simulink model "NandiniG_23EEM1S02_foc_5mli_working_fine_Cap"  (R2024b)
settings: Solver=ode1  StartTime=0.0  StopTime=1  FixedStep=0.000001  MaxStep=1e-4  RelTol=1e-3
model workspace (MAT data in the model file):
  Vdcref = 40
  Vref = 450
  fs = 2054
  k = 1
  ma = 1
undefined symbols (not defined in the file): Kcq, Kcs
libraries: spsIGBTDiodeLib x28, simulink x20, spsDiodeLib x18, spsVoltageMeasurementLib x12, slpidlib x9, spsSeriesRLCBranchLib x8, powerlib_extras x3, spsCurrentMeasurementLib x3, spsDCVoltageSourceLib x1, spsGroundLib x1, spsPermanentMagnetSynchronousMachineLib x1, spsThreePhaseVIMeasurementLib x1
(part 2 of 2)

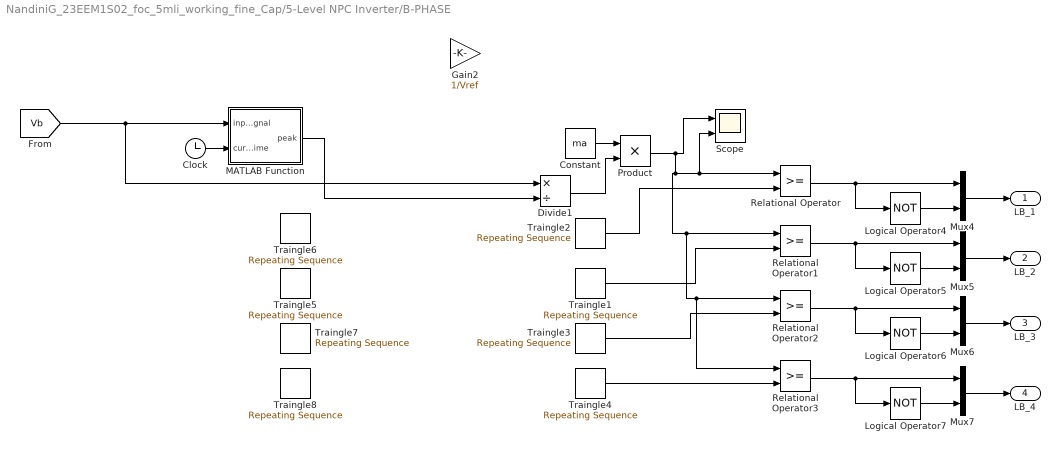
== system NandiniG_23EEM1S02_foc_5mli_working_fine_Cap/5-Level NPC Inverter/B-PHASE ==
  Clock : Clock
  Constant : Constant  Value=ma
  Divide1 : Product  Inputs=*/
  Gain2 : Gain  Gain=1/Vref
  Logical Operator{4..7} (4 alike) : Logic  Operator=NOT  AllPortsSameDT=off  OutDataTypeStr=boolean
  MATLAB Function : MATLAB Function  TreatAsAtomicUnit=on
  Mux{4..7} (4 alike) : Mux  Inputs=2
  Product : Product
  Relational Operator{,1..3} (4 alike) : RelationalOperator  OutDataTypeStr=boolean  InputSameDT=off
  Scope : Scope  NumInputPorts=2
  Traingle1 : simulink/Sources/Repeating Sequence  rep_seq_t=[0 0.25/fs 0.5/fs 0.75/fs 1/fs]  rep_seq_y=[0 0.25 0.5 0.25 0]*k
  Traingle2 : simulink/Sources/Repeating Sequence  rep_seq_t=[0 0.25/fs 0.5/fs 0.75/fs 1/fs]  rep_seq_y="[0.5 0.75 1 0.75  0.5]*k"
  Traingle3 : simulink/Sources/Repeating Sequence  rep_seq_t=[0 0.25/fs 0.5/fs 0.75/fs 1/fs]  rep_seq_y=[-0.5 -0.25 0 -0.25 -0.5]*k
  Traingle4 : simulink/Sources/Repeating Sequence  rep_seq_t=[0 0.25/fs 0.5/fs 0.75/fs 1/fs]  rep_seq_y=[-1 -0.75 -0.5 -0.75 -1]*k
  Traingle5 : simulink/Sources/Repeating Sequence  rep_seq_t=[0 0.25/fs 0.5/fs 0.75/fs 1/fs]  rep_seq_y=[565*0.25 565/2 565*0.25 0 565*0.25]
  Traingle6 : simulink/Sources/Repeating Sequence  rep_seq_t=[0 0.25/fs 0.5/fs 0.75/fs 1/fs]  rep_seq_y=[565*0.75 565 565*0.75 565/2 565*0.75]
  Traingle7 : simulink/Sources/Repeating Sequence  rep_seq_t=[0 0.25/fs 0.5/fs 0.75/fs 1/fs]  rep_seq_y=[-565*0.25 0 -565*0.25 -565/2 -565*0.25]
  Traingle8 : simulink/Sources/Repeating Sequence  rep_seq_t=[0 0.25/fs 0.5/fs 0.75/fs 1/fs]  rep_seq_y=[-565*0.75 -565/2 -565*0.75 -565 -565*0.75]
  LB_1 : Outport
  LB_2 : Outport  Port=2
  LB_3 : Outport  Port=3
  LB_4 : Outport  Port=4
  wires:
  Relational Operator/1 -> Logical Operator4/1, Mux4/1
  Logical Operator4/1 -> Mux4/2
  Mux4/1 -> LB_1/1
  Relational Operator1/1 -> Mux5/1, Logical Operator5/1
  Logical Operator5/1 -> Mux5/2
  Mux5/1 -> LB_2/1
  Relational Operator2/1 -> Logical Operator6/1, Mux6/1
  Logical Operator6/1 -> Mux6/2
  Mux6/1 -> LB_3/1
  Relational Operator3/1 -> Mux7/1, Logical Operator7/1
  Logical Operator7/1 -> Mux7/2
  Mux7/1 -> LB_4/1
  Traingle1/1 -> Relational Operator1/2
  Traingle2/1 -> Relational Operator/2
  Traingle4/1 -> Relational Operator3/2
  Traingle3/1 -> Relational Operator2/2
  [Vb] -> MATLAB Function/1(inputSignal), Divide1/1
  MATLAB Function/1(peak) -> Divide1/2
  Divide1/1 -> Product/2
  Constant/1 -> Product/1
  Product/1 -> Relational Operator3/1, Relational Operator2/1, Relational Operator1/1, Scope/2, Relational Operator/1, Scope/1
  Clock/1 -> MATLAB Function/2(currentTime)

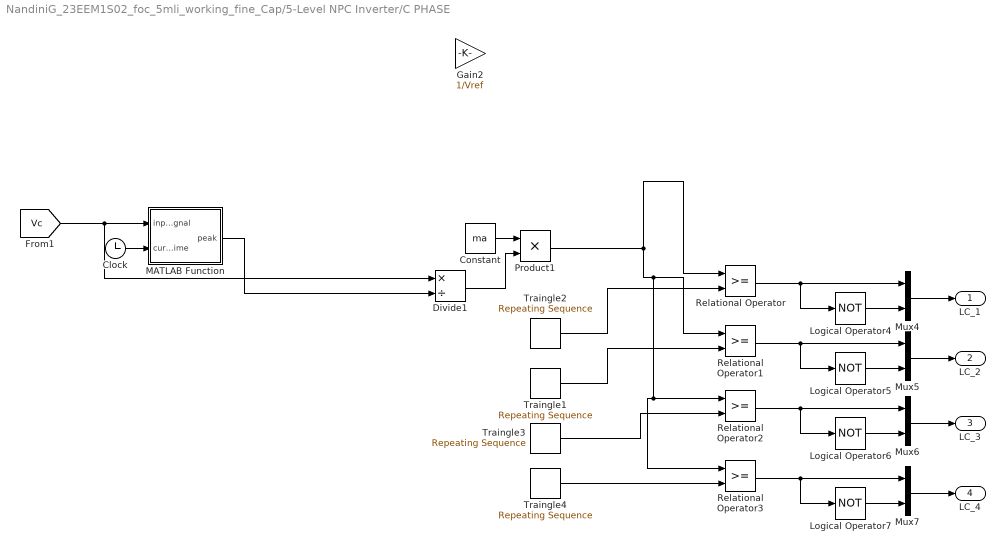
== system NandiniG_23EEM1S02_foc_5mli_working_fine_Cap/5-Level NPC Inverter/C PHASE ==
  Clock : Clock
  Constant : Constant  Value=ma
  Divide1 : Product  Inputs=*/
  Gain2 : Gain  Gain=1/Vref
  Logical Operator{4..7} (4 alike) : Logic  Operator=NOT  AllPortsSameDT=off  OutDataTypeStr=boolean
  MATLAB Function : MATLAB Function  TreatAsAtomicUnit=on
  Mux{4..7} (4 alike) : Mux  Inputs=2
  Product1 : Product
  Relational Operator{,1..3} (4 alike) : RelationalOperator  OutDataTypeStr=boolean  InputSameDT=off
  Traingle1 : simulink/Sources/Repeating Sequence  rep_seq_t=[0 0.25/fs 0.5/fs 0.75/fs 1/fs]  rep_seq_y=[0 0.25 0.5 0.25 0]*k
  Traingle2 : simulink/Sources/Repeating Sequence  rep_seq_t=[0 0.25/fs 0.5/fs 0.75/fs 1/fs]  rep_seq_y="[0.5 0.75 1 0.75  0.5]*k"
  Traingle3 : simulink/Sources/Repeating Sequence  rep_seq_t=[0 0.25/fs 0.5/fs 0.75/fs 1/fs]  rep_seq_y=[-0.5 -0.25 0 -0.25 -0.5]*k
  Traingle4 : simulink/Sources/Repeating Sequence  rep_seq_t=[0 0.25/fs 0.5/fs 0.75/fs 1/fs]  rep_seq_y=[-1 -0.75 -0.5 -0.75 -1]*k
  LC_1 : Outport
  LC_2 : Outport  Port=2
  LC_3 : Outport  Port=3
  LC_4 : Outport  Port=4
  wires:
  Mux7/1 -> LC_4/1
  Logical Operator7/1 -> Mux7/2
  Relational Operator3/1 -> Logical Operator7/1, Mux7/1
  Mux6/1 -> LC_3/1
  Logical Operator6/1 -> Mux6/2
  Relational Operator2/1 -> Mux6/1, Logical Operator6/1
  Mux5/1 -> LC_2/1
  Logical Operator5/1 -> Mux5/2
  Relational Operator1/1 -> Logical Operator5/1, Mux5/1
  Mux4/1 -> LC_1/1
  Logical Operator4/1 -> Mux4/2
  Relational Operator/1 -> Mux4/1, Logical Operator4/1
  Traingle1/1 -> Relational Operator1/2
  Traingle2/1 -> Relational Operator/2
  Traingle4/1 -> Relational Operator3/2
  Traingle3/1 -> Relational Operator2/2
  MATLAB Function/1(peak) -> Divide1/2
  Divide1/1 -> Product1/2
  Constant/1 -> Product1/1
  [Vc] -> MATLAB Function/1(inputSignal), Divide1/1
  Product1/1 -> Relational Operator/1, Relational Operator1/1, Relational Operator3/1, Relational Operator2/1
  Clock/1 -> MATLAB Function/2(currentTime)

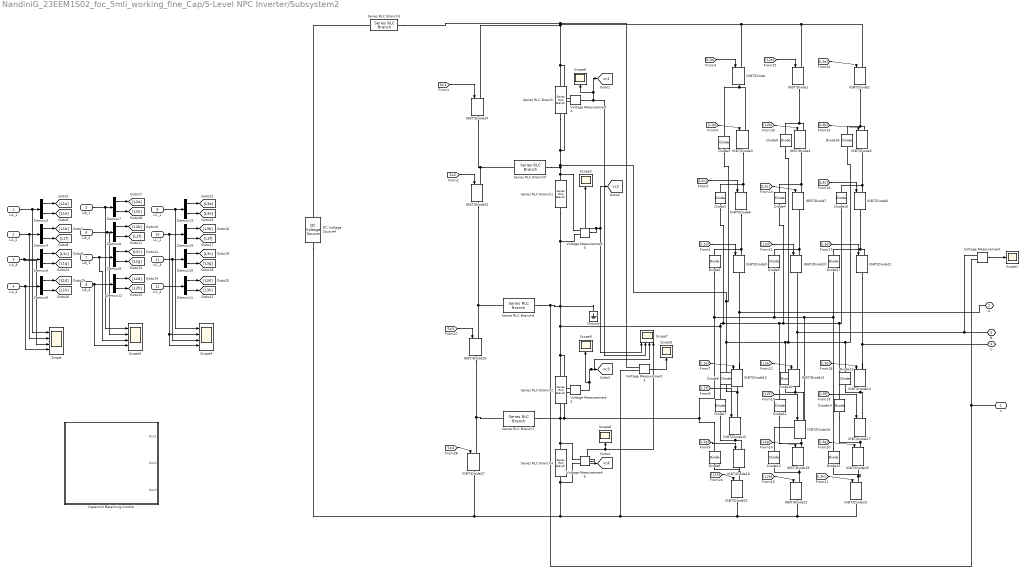
== system NandiniG_23EEM1S02_foc_5mli_working_fine_Cap/5-Level NPC Inverter/Subsystem2 ==
  LA_1 : Inport
  LA_2 : Inport  Port=2
  LA_3 : Inport  Port=3
  LA_4 : Inport  Port=4
  LB_1 : Inport  Port=5
  LB_2 : Inport  Port=6
  LB_3 : Inport  Port=7
  LB_4 : Inport  Port=8
  LC_1 : Inport  Port=9
  LC_2 : Inport  Port=10
  LC_3 : Inport  Port=11
  LC_4 : Inport  Port=12
  " Capacitor Balancing Control" : Subsystem
  DC Voltage Source4 : spsDCVoltageSourceLib/DC Voltage Source  Amplitude=160  Measurements=None
  Demux{3..14} (12 alike) : Demux  Outputs=2
  Diode{1..18} (18 alike) : spsDiodeLib/Diode  Ron=0.001  Lon=0  Vf=0.8  IC=0  UseSnubber=off  Rs=500  Cs=250e-9  Measurements=off
  Ground : spsGroundLib/Ground  LConnTagsString=a
  IGBT/Diode{,1..27} (28 alike) : spsIGBTDiodeLib/IGBT//Diode  Ron=1e-3  Rs=1e5  Cs=inf  Measurements=off
  Scope{,3..4,7} (4 alike) : Scope  NumInputPorts=4
  Scope{1..2,5..6,8..9} (6 alike) : Scope
  Series RLC Branch{,1..2,4} (4 alike) : spsSeriesRLCBranchLib/Series RLC Branch  LConnTagsString=__new0  RConnTagsString=__new0  BranchType=C  Resistance=1  Inductance=1e-3  SetiL0=off  InitialCurrent=0  Capacitance=4500e-6  Setx0=on  InitialVoltage=Vdcref  Measurements=None
  Series RLC Branch3 : spsSeriesRLCBranchLib/Series RLC Branch  LConnTagsString=__new0  RConnTagsString=__new0  BranchType=R  Resistance=0.001  Inductance=1e-3  SetiL0=off  InitialCurrent=0  Capacitance=1e-6  Setx0=off  InitialVoltage=0  Measurements=None
  Series RLC Branch5 : spsSeriesRLCBranchLib/Series RLC Branch  LConnTagsString=__new0  RConnTagsString=__new0  BranchType=RL  Resistance=1  Inductance=1e-3  SetiL0=off  InitialCurrent=0  Capacitance=1e-6  Setx0=off  InitialVoltage=0  Measurements=None
  Series RLC Branch6 : spsSeriesRLCBranchLib/Series RLC Branch  LConnTagsString=__new0  RConnTagsString=__new0  BranchType=RL  Resistance=1  Inductance=1e-3  SetiL0=off  InitialCurrent=0  Capacitance=1e-6  Setx0=off  InitialVoltage=0  Measurements=None
  Series RLC Branch7 : spsSeriesRLCBranchLib/Series RLC Branch  LConnTagsString=__new0  RConnTagsString=__new0  BranchType=RL  Resistance=1  Inductance=1e-3  SetiL0=off  InitialCurrent=0  Capacitance=1e-6  Setx0=off  InitialVoltage=0  Measurements=None
  Voltage Measurement{,2..6} (6 alike) : spsVoltageMeasurementLib/Voltage Measurement  PhasorSimulation=off  OutputType=Complex  PSBequivalent=0
  " n" : PMIOPort  Side=Right
  A : PMIOPort  Port=2  Side=Right
  B : PMIOPort  Port=3  Side=Right
  C : PMIOPort  Port=4  Side=Right
  tag scope: vc1=global, vc2=global, vc3=global, vc4=global
  wires:
  Demux5/1 -> [L1c]
  [L1a] -> IGBT/Diode/1
  Demux13/2 -> [L3e]
  Demux9/2 -> [L2g]
  Demux6/1 -> [L1d]
  Demux13/1 -> [L3a]
  [L3b] -> IGBT/Diode5/1
  Demux12/2 -> [L2h]
  [L3h] -> IGBT/Diode23/1
  LB_4/1 -> Demux12/1, Scope3/4
  [L1h] -> IGBT/Diode21/1
  Demux8/1 -> [L2b]
  [L3f] -> IGBT/Diode17/1
  LA_3/1 -> Scope/3, Demux5/1
  Demux14/1 -> [L3b]
  [L2f] -> IGBT/Diode16/1
  Demux3/2 -> [L1e]
  [L2d] -> IGBT/Diode10/1
  LC_2/1 -> Scope4/4, Scope4/2, Demux14/1
  Demux10/1 -> [L3c]
  LB_1/1 -> Scope3/1, Demux7/1
  LB_3/1 -> Scope3/3, Demux9/1
  Demux7/2 -> [L2e]
  Demux12/1 -> [L2d]
  Demux11/1 -> [L3d]
  [L2a] -> IGBT/Diode1/1
  LC_1/1 -> Scope4/1, Demux13/1
  [L2b] -> IGBT/Diode4/1
  [L3e] -> IGBT/Diode14/1
  LA_1/1 -> Scope/1, Demux3/1
  [L2h] -> IGBT/Diode22/1
  Demux3/1 -> [L1a]
  Demux6/2 -> [L1h]
  [L1e] -> IGBT/Diode12/1
  Demux9/1 -> [L2c]
  [L3d] -> IGBT/Diode11/1
  [L1f] -> IGBT/Diode15/1
  Demux4/1 -> [L1b]
  [L2e] -> IGBT/Diode13/1
  [L3c] -> IGBT/Diode8/1
  [L2g] -> IGBT/Diode19/1
  Demux5/2 -> [L1g]
  Demux10/2 -> [L3g]
  LA_2/1 -> Demux4/1, Scope/2
  LC_3/1 -> Scope4/3, Demux10/1
  [L2c] -> IGBT/Diode7/1
  Demux7/1 -> [L2a]
  [L1g] -> IGBT/Diode18/1
  [L1d] -> IGBT/Diode9/1
  LC_4/1 -> Demux11/1
  [L1c] -> IGBT/Diode6/1
  [L1b] -> IGBT/Diode3/1
  Demux11/2 -> [L3h]
  LB_2/1 -> Scope3/2, Demux8/1
  [L3a] -> IGBT/Diode2/1
  Demux4/2 -> [L1f]
  Demux8/2 -> [L2f]
  LA_4/1 -> Scope/4, Demux6/1
  Demux14/2 -> [L3f]
  [L3g] -> IGBT/Diode20/1
  Voltage Measurement/1 -> Scope1/1
  Voltage Measurement5/1 -> [vc2], Scope7/1, Scope2/1
  Voltage Measurement3/1 -> Scope5/1
  Voltage Measurement4/1 -> Scope7/2, Scope6/1, [vc1]
  Voltage Measurement2/1 -> Scope9/1, Scope7/3, [vc3]
  Voltage Measurement6/1 -> [vc4], Scope7/4, Scope8/1
  [Sc1] -> IGBT/Diode24/1
  [Sc2] -> IGBT/Diode25/1
  [Sc3] -> IGBT/Diode26/1
  [Sc4] -> IGBT/Diode27/1
  connections:
  IGBT/Diode20/LConn1 -- IGBT/Diode17/RConn1 -- Diode14/LConn1
  IGBT/Diode7/LConn1 -- IGBT/Diode4/RConn1 -- Diode4/RConn1
  IGBT/Diode3/LConn1 -- IGBT/Diode/RConn1 -- Diode3/RConn1
  Diode10/LConn1 -- IGBT/Diode13/RConn1 -- IGBT/Diode16/LConn1
  IGBT/Diode17/LConn1 -- IGBT/Diode14/RConn1 -- Diode13/LConn1
  Voltage Measurement5/LConn1 -- Series RLC Branch/RConn1 -- Voltage Measurement4/LConn2 -- Diode9/LConn1 -- Diode18/LConn1 -- Diode13/RConn1 -- Diode10/RConn1 -- Diode6/RConn1 -- Diode3/LConn1 -- Series RLC Branch5/RConn1 -- Series RLC Branch1/LConn1
  Diode9/RConn1 -- IGBT/Diode1/RConn1 -- IGBT/Diode4/LConn1
  IGBT/Diode5/RConn1 -- IGBT/Diode8/LConn1 -- Diode16/RConn1
  IGBT/Diode11/RConn1 -- IGBT/Diode14/LConn1 -- C/RConn1
  Series RLC Branch4/RConn1 -- IGBT/Diode27/RConn1 -- DC Voltage Source4/LConn1 -- Voltage Measurement3/LConn2 -- IGBT/Diode21/RConn1 -- IGBT/Diode23/RConn1 -- IGBT/Diode22/RConn1 -- Voltage Measurement6/LConn2
  IGBT/Diode15/RConn1 -- IGBT/Diode18/LConn1 -- Diode7/LConn1
  Diode8/LConn1 -- IGBT/Diode18/RConn1 -- IGBT/Diode21/LConn1
  IGBT/Diode26/RConn1 -- Series RLC Branch7/LConn1 -- IGBT/Diode27/LConn1
  IGBT/Diode16/RConn1 -- Diode11/LConn1 -- IGBT/Diode19/LConn1
  IGBT/Diode7/RConn1 -- IGBT/Diode10/LConn1 -- Diode5/RConn1
  IGBT/Diode2/RConn1 -- Diode18/RConn1 -- IGBT/Diode5/LConn1
  Voltage Measurement4/LConn1 -- Voltage Measurement3/LConn1 -- Series RLC Branch3/LConn1 -- IGBT/Diode/LConn1 -- IGBT/Diode1/LConn1 -- IGBT/Diode2/LConn1 -- IGBT/Diode24/LConn1 -- Series RLC Branch/LConn1
  IGBT/Diode6/LConn1 -- IGBT/Diode3/RConn1 -- Diode1/RConn1
  IGBT/Diode22/LConn1 -- IGBT/Diode19/RConn1 -- Diode12/LConn1
  Voltage Measurement/LConn1 -- IGBT/Diode13/LConn1 -- IGBT/Diode10/RConn1 -- B/RConn1
  IGBT/Diode12/RConn1 -- Diode6/LConn1 -- IGBT/Diode15/LConn1
  IGBT/Diode12/LConn1 -- IGBT/Diode9/RConn1 -- A/RConn1
  Diode15/LConn1 -- IGBT/Diode20/RConn1 -- IGBT/Diode23/LConn1
  Diode17/RConn1 -- IGBT/Diode8/RConn1 -- IGBT/Diode11/LConn1
  IGBT/Diode9/LConn1 -- Diode2/RConn1 -- IGBT/Diode6/RConn1
  IGBT/Diode25/RConn1 -- IGBT/Diode26/LConn1 -- Series RLC Branch6/LConn1
  DC Voltage Source4/RConn1 -- Series RLC Branch3/RConn1
  IGBT/Diode24/RConn1 -- Series RLC Branch5/LConn1 -- IGBT/Diode25/LConn1
  Diode1/LConn1 -- Diode7/RConn1 -- Voltage Measurement/LConn2 -- " n"/RConn1 -- Series RLC Branch6/RConn1 -- Ground/LConn1 -- Series RLC Branch1/RConn1 -- Voltage Measurement5/LConn2 -- Series RLC Branch2/LConn1 -- Voltage Measurement2/LConn1 -- Diode4/LConn1 -- Diode16/LConn1 -- Diode14/RConn1 -- Diode11/RConn1
  Series RLC Branch2/RConn1 -- Series RLC Branch7/RConn1 -- Voltage Measurement6/LConn1 -- Series RLC Branch4/LConn1 -- Diode2/LConn1 -- Diode5/LConn1 -- Diode17/LConn1 -- Diode15/RConn1 -- Diode12/RConn1 -- Diode8/RConn1 -- Voltage Measurement2/LConn2

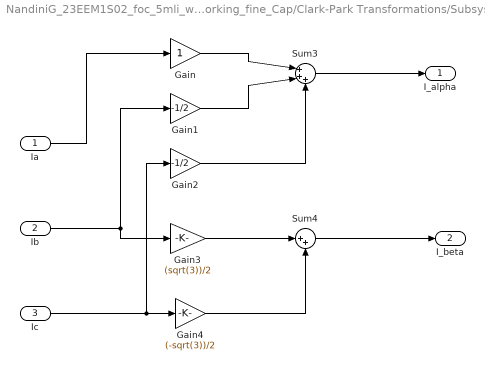
== system NandiniG_23EEM1S02_foc_5mli_working_fine_Cap/Clark-Park Transformations/Subsystem ==
  Ia : Inport
  Ib : Inport  Port=2
  Ic : Inport  Port=3
  Gain : Gain
  Gain1 : Gain  Gain=-1/2
  Gain2 : Gain  Gain=-1/2
  Gain3 : Gain  Gain=(sqrt(3))/2
  Gain4 : Gain  Gain=(-sqrt(3))/2
  Sum3 : Sum  Inputs=|+++
  Sum4 : Sum  Inputs=|++
  I_alpha : Outport
  I_beta : Outport  Port=2
  wires:
  Gain2/1 -> Sum3/3
  Ib/1 -> Gain3/1, Gain1/1
  Sum3/1 -> I_alpha/1
  Gain3/1 -> Sum4/1
  Gain/1 -> Sum3/1
  Ic/1 -> Gain4/1, Gain2/1
  Gain1/1 -> Sum3/2
  Gain4/1 -> Sum4/2
  Ia/1 -> Gain/1
  Sum4/1 -> I_beta/1

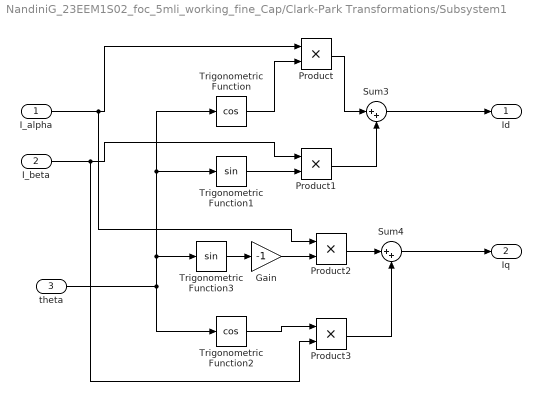
== system NandiniG_23EEM1S02_foc_5mli_working_fine_Cap/Clark-Park Transformations/Subsystem1 ==
  I_alpha : Inport
  I_beta : Inport  Port=2
  theta : Inport  Port=3
  Gain : Gain  Gain=-1
  Product{,1..3} (4 alike) : Product
  Sum3 : Sum  Inputs=|++
  Sum4 : Sum  Inputs=|++
  Trigonometric Function : Trigonometry  Operator=cos
  Trigonometric Function1 : Trigonometry
  Trigonometric Function2 : Trigonometry  Operator=cos
  Trigonometric Function3 : Trigonometry
  Id : Outport
  Iq : Outport  Port=2
  wires:
  Sum3/1 -> Id/1
  Sum4/1 -> Iq/1
  Trigonometric Function3/1 -> Gain/1
  theta/1 -> Trigonometric Function2/1, Trigonometric Function3/1, Trigonometric Function1/1, Trigonometric Function/1
  Trigonometric Function/1 -> Product/2
  I_alpha/1 -> Product2/1, Product/1
  Trigonometric Function1/1 -> Product1/2
  I_beta/1 -> Product3/2, Product1/1
  Product/1 -> Sum3/1
  Product1/1 -> Sum3/2
  Gain/1 -> Product2/2
  Trigonometric Function2/1 -> Product3/1
  Product2/1 -> Sum4/1
  Product3/1 -> Sum4/2

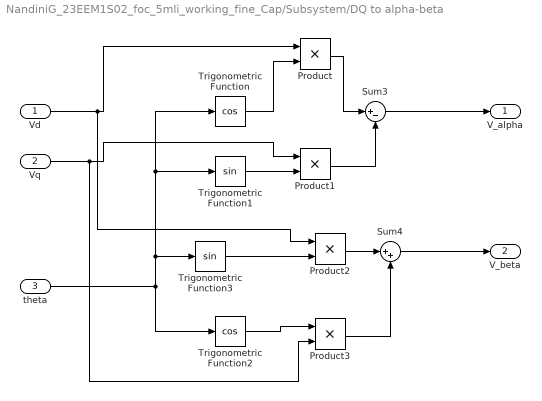
== system NandiniG_23EEM1S02_foc_5mli_working_fine_Cap/Subsystem/DQ to alpha-beta ==
  Vd : Inport
  Vq : Inport  Port=2
  theta : Inport  Port=3
  Product{,1..3} (4 alike) : Product
  Sum3 : Sum  Inputs=|+-
  Sum4 : Sum  Inputs=|++
  Trigonometric Function : Trigonometry  Operator=cos
  Trigonometric Function1 : Trigonometry
  Trigonometric Function2 : Trigonometry  Operator=cos
  Trigonometric Function3 : Trigonometry
  V_alpha : Outport
  V_beta : Outport  Port=2
  wires:
  Product3/1 -> Sum4/2
  Product2/1 -> Sum4/1
  Trigonometric Function2/1 -> Product3/1
  Trigonometric Function3/1 -> Product2/2
  Product1/1 -> Sum3/2
  Product/1 -> Sum3/1
  Vq/1 -> Product1/1, Product3/2
  Trigonometric Function1/1 -> Product1/2
  Vd/1 -> Product/1, Product2/1
  Trigonometric Function/1 -> Product/2
  theta/1 -> Trigonometric Function/1, Trigonometric Function1/1, Trigonometric Function3/1, Trigonometric Function2/1
  Sum4/1 -> V_beta/1
  Sum3/1 -> V_alpha/1

== system NandiniG_23EEM1S02_foc_5mli_working_fine_Cap/Subsystem/alpha-beta to ABC ==
  alpha_beta : Inport
  Demux : Demux  Outputs=2
  Gain5 : Gain  Gain=2/3
  Gain6 : Gain  Gain=1/sqrt(3)
  Gain7 : Gain  Gain=-1/3
  Gain8 : Gain  Gain=-1/3
  Gain9 : Gain  Gain=-1/sqrt(3)
  Sum1 : Sum  Inputs=|++
  Sum2 : Sum  Inputs=|++
  Va : Outport
  Vb : Outport  Port=2
  Vc : Outport  Port=3
  wires:
  Demux/1 -> Gain5/1, Gain8/1, Gain7/1
  Gain5/1 -> Va/1
  Demux/2 -> Gain9/1, Gain6/1
  Gain6/1 -> Sum1/1
  Gain7/1 -> Sum1/2
  Sum1/1 -> Vb/1
  Gain8/1 -> Sum2/1
  Gain9/1 -> Sum2/2
  Sum2/1 -> Vc/1
  alpha_beta/1 -> Demux/1

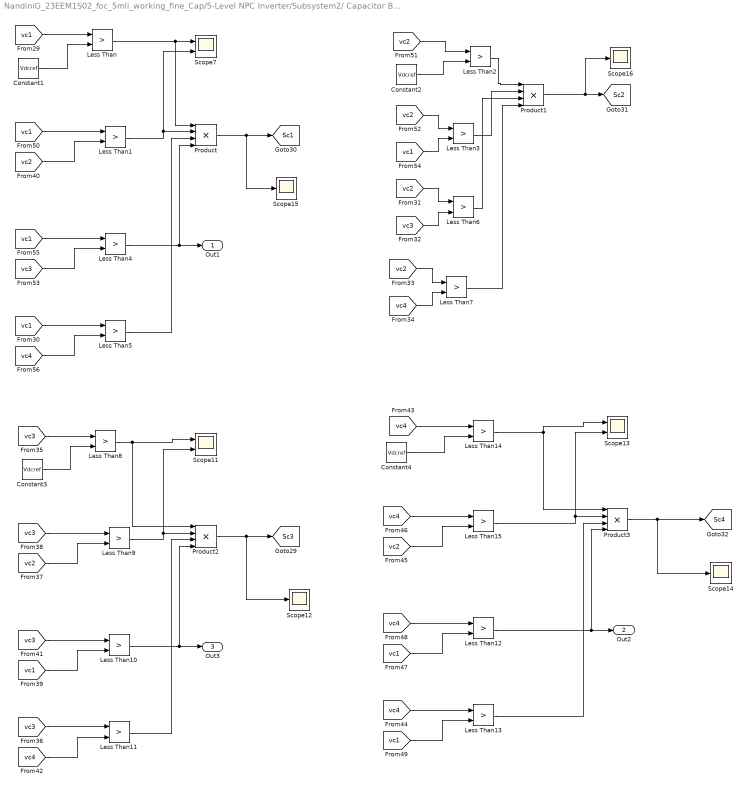
== system NandiniG_23EEM1S02_foc_5mli_working_fine_Cap/5-Level NPC Inverter/Subsystem2/ Capacitor Balancing Control ==
  Constant{1..4} (4 alike) : Constant  Value=Vdcref
  Less Than{,1..15} (16 alike) : RelationalOperator  Operator=>  OutDataTypeStr=boolean  RndMeth=Simplest  InputSameDT=off
  Product{,1..3} (4 alike) : Product  Inputs=4
  Scope11 : Scope  NumInputPorts=2
  Scope{12,14..16} (4 alike) : Scope
  Scope13 : Scope  NumInputPorts=2
  Scope7 : Scope  NumInputPorts=2
  Out1 : Outport
  Out2 : Outport  Port=2
  Out3 : Outport  Port=3
  tag scope: Sc1=global, Sc2=global, Sc3=global, Sc4=global
  wires:
  [vc1] -> Less Than5/1
  [vc1] -> Less Than1/1
  Less Than12/1 -> Out2/1, Product3/4
  Product2/1 -> [Sc3], Scope12/1
  Product/1 -> Scope15/1, [Sc1]
  Constant2/1 -> Less Than2/2
  [vc3] -> Less Than10/1
  Less Than3/1 -> Product1/2
  Less Than15/1 -> Scope13/2, Product3/2
  Less Than9/1 -> Product2/2, Scope11/2
  [vc1] -> Less Than/1
  [vc1] -> Less Than13/2
  [vc4] -> Less Than13/1
  Product1/1 -> Scope16/1, [Sc2]
  [vc3] -> Less Than4/2
  Less Than2/1 -> Product1/1
  Less Than13/1 -> Product3/3
  [vc2] -> Less Than15/2
  [vc1] -> Less Than3/2
  Less Than7/1 -> Product1/4
  [vc1] -> Less Than12/2
  Constant1/1 -> Less Than/2
  Less Than11/1 -> Product2/3
  Less Than14/1 -> Scope13/1, Product3/1
  [vc2] -> Less Than3/1
  [vc2] -> Less Than9/2
  Product3/1 -> Scope14/1, [Sc4]
  [vc4] -> Less Than7/2
  Constant4/1 -> Less Than14/2
  [vc4] -> Less Than11/2
  [vc4] -> Less Than12/1
  [vc1] -> Less Than4/1
  [vc3] -> Less Than9/1
  [vc2] -> Less Than2/1
  [vc4] -> Less Than15/1
  [vc4] -> Less Than5/2
  Less Than4/1 -> Out1/1, Product/4
  [vc3] -> Less Than8/1
  [vc2] -> Less Than6/1
  [vc2] -> Less Than7/1
  [vc1] -> Less Than10/2
  Less Than6/1 -> Product1/3
  [vc3] -> Less Than6/2
  [vc4] -> Less Than14/1
  Less Than5/1 -> Product/3
  Less Than1/1 -> Scope7/2, Product/2
  Less Than/1 -> Product/1, Scope7/1
  Less Than8/1 -> Scope11/1, Product2/1
  Constant3/1 -> Less Than8/2
  [vc3] -> Less Than11/1
  Less Than10/1 -> Out3/1, Product2/4
  [vc2] -> Less Than1/2

== matlab function NandiniG_23EEM1S02_foc_5mli_working_fine_Cap/5-Level NPC Inverter/B-PHASE/MATLAB Function ==
  settings: updateMethod=DISCRETE
  data: inputSignal input; peak output; currentTime input
function peak = getPeak(inputSignal, currentTime)
    % GETPEAK Function to track the peak value of a running waveform.
    %
    % INPUT:
    % inputSignal - Current sample of the waveform.
    % currentTime - Current simulation time.
    %
    % OUTPUT:
    % peak - The maximum absolute value encountered so far.
 
    % Persistent variables to store the peak values and the reset flag
    persistent maxPeak minPeak resetDone;
 
    % Initialize the persistent variables on the first function call
    if isempty(maxPeak)
        maxPeak = -inf;  % Start with a very low value
    end
    if isempty(minPeak)
        minPeak = inf;   % Start with a very high value
    end
    if isempty(resetDone)
        resetDone = false;  % Flag to indicate if reset has been done
    end
 
    % Reset the peak values once at 0.1 seconds
    if currentTime >= 0.11 && ~resetDone
        maxPeak = -inf;
        minPeak = inf;
        resetDone = true;  % Set the flag to true after reset
    end
 
    % Update the peak values if the current sample is larger or smaller
    if inputSignal > maxPeak
        maxPeak = inputSignal;
    end
    if inputSignal < minPeak
        minPeak = inputSignal;
    end
 
    % Calculate the peak-to-peak value
    peak = max(abs(maxPeak), abs(minPeak));
end

== matlab function NandiniG_23EEM1S02_foc_5mli_working_fine_Cap/5-Level NPC Inverter/A-PHASE/MATLAB Function ==
  settings: updateMethod=DISCRETE
  data: inputSignal input; peak output; currentTime input
function peak = getPeak(inputSignal, currentTime)
    % GETPEAK Function to track the peak value of a running waveform.
    %
    % INPUT:
    % inputSignal - Current sample of the waveform.
    % currentTime - Current simulation time.
    %
    % OUTPUT:
    % peak - The maximum absolute value encountered so far.
 
    % Persistent variables to store the peak values and the reset flag
    persistent maxPeak minPeak resetDone;
 
    % Initialize the persistent variables on the first function call
    if isempty(maxPeak)
        maxPeak = -inf;  % Start with a very low value
    end
    if isempty(minPeak)
        minPeak = inf;   % Start with a very high value
    end
    if isempty(resetDone)
        resetDone = false;  % Flag to indicate if reset has been done
    end
 
    % Reset the peak values once at 0.1 seconds
    if currentTime >= 0.11 && ~resetDone
        maxPeak = -inf;
        minPeak = inf;
        resetDone = true;  % Set the flag to true after reset
    end
 
    % Update the peak values if the current sample is larger or smaller
    if inputSignal > maxPeak
        maxPeak = inputSignal;
    end
    if inputSignal < minPeak
        minPeak = inputSignal;
    end
 
    % Calculate the peak-to-peak value
    peak = max(abs(maxPeak), abs(minPeak));
end

== matlab function NandiniG_23EEM1S02_foc_5mli_working_fine_Cap/5-Level NPC Inverter/C PHASE/MATLAB Function ==
  settings: updateMethod=DISCRETE
  data: inputSignal input; peak output; currentTime input
function peak = getPeak(inputSignal, currentTime)
    % GETPEAK Function to track the peak value of a running waveform.
    %
    % INPUT:
    % inputSignal - Current sample of the waveform.
    % currentTime - Current simulation time.
    %
    % OUTPUT:
    % peak - The maximum absolute value encountered so far.
 
    % Persistent variables to store the peak values and the reset flag
    persistent maxPeak minPeak resetDone;
 
    % Initialize the persistent variables on the first function call
    if isempty(maxPeak)
        maxPeak = -inf;  % Start with a very low value
    end
    if isempty(minPeak)
        minPeak = inf;   % Start with a very high value
    end
    if isempty(resetDone)
        resetDone = false;  % Flag to indicate if reset has been done
    end
 
    % Reset the peak values once at 0.1 seconds
    if currentTime >= 0.11 && ~resetDone
        maxPeak = -inf;
        minPeak = inf;
        resetDone = true;  % Set the flag to true after reset
    end
 
    % Update the peak values if the current sample is larger or smaller
    if inputSignal > maxPeak
        maxPeak = inputSignal;
    end
    if inputSignal < minPeak
        minPeak = inputSignal;
    end
 
    % Calculate the peak-to-peak value
    peak = max(abs(maxPeak), abs(minPeak));
end
